simulink model "shuntDCmotor"  (R2018a)
settings: Solver=VariableStepAuto  StartTime=0.0  StopTime=10  RelTol=1e-3
values from neighbouring files (symbols this model uses):
  Bm = 0.00000604    (= 6.04e-06)    [PMDCparameters.m]    (also in SEDCparameters.m = 1.074e-06; SeriseDCparameters.m = 0.0025; ShuntDCparameters.m = 1.074e-06)
  J = 0.00000161    (= 1.61e-06)    [PMDCparameters.m]    (also in SEDCparameters.m = 0.21; SeriseDCparameters.m = 0.02365; ShuntDCparameters.m = 0.21)
  LAA = 0.12    [PMDCparameters.m]    (also in SEDCparameters.m = 0.01; SeriseDCparameters.m; ShuntDCparameters.m = 0.01)
  LAF = 0.004    [SEDCparameters.m]    (also in SeriseDCparameters.m = 0.0675; ShuntDCparameters.m)
  LFF = 0.167    [SEDCparameters.m]    (also in SeriseDCparameters.m = 0.03; ShuntDCparameters.m)
  ra = 7    [PMDCparameters.m]    (also in SEDCparameters.m = 0.013; SeriseDCparameters.m = 1.5; ShuntDCparameters.m = 0.013)
  rf = 1.43    [SEDCparameters.m]    (also in SeriseDCparameters.m = 0.7; ShuntDCparameters.m)
  Tl = 0.003    [PMDCparameters.m]    (also in SEDCparameters.m = 2.493; SeriseDCparameters.m = 10; ShuntDCparameters.m = 2.493)
  Va = 6    [PMDCparameters.m]    (also in SEDCparameters.m = 24; SeriseDCparameters.m = 100; ShuntDCparameters.m = 24)
libraries: fl_lib x15, nesl_utility x10, powerlib x3
settings Model: Creator=Noor  LastModifiedBy=Noor

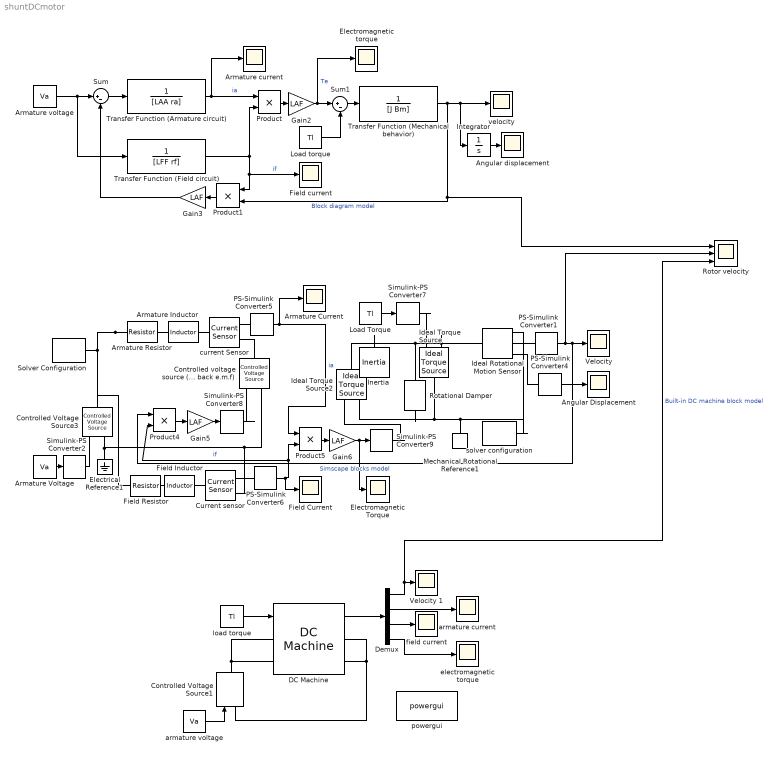
== system shuntDCmotor ==
  " Ideal Torque Source" : fl_lib/Mechanical/Mechanical Sources/Ideal Torque Source
  Angular Displacement : Scope
  Angular displacement : Scope
  Armature Voltage : Constant  Value=Va
  Armature Inductor : fl_lib/Electrical/Electrical Elements/Inductor  l=LAA H  r=0 Ohm  g=0 1/Ohm  i_specify=off  i_priority=None  i=0 A  i_nominal_specify=off  i_nominal_unit=A  i_nominal_value=1  v_specify=off  v_priority=None  v=0 V  v_nominal_specify=off  v_nominal_unit=V  v_nominal_value=1  i_L_specify=off  i_L_priority=High  i_L=0 A  i_L_nominal_specify=off  i_L_nominal_unit=A  i_L_nominal_value=1
  Armature Resistor : fl_lib/Electrical/Electrical Elements/Resistor  R=ra Ohm  i_specify=off  i_priority=None  i=0 A  i_nominal_specify=off  i_nominal_unit=A  i_nominal_value=1  v_specify=off  v_priority=None  v=0 V  v_nominal_specify=off  v_nominal_unit=V  v_nominal_value=1
  Armature Current : Scope
  Armature current : Scope
  Armature voltage : Constant  Value=Va
  Controlled voltage source (i.e. back e.m.f) : fl_lib/Electrical/Electrical Sources/Controlled Voltage Source
  Controlled Voltage Source3 : fl_lib/Electrical/Electrical Sources/Controlled Voltage Source
  Controlled Voltage Source1 : powerlib/Electrical Sources/Controlled Voltage Source  Initialize=on  Source_Type=AC  Amplitude=0  Phase=0  Frequency=0  Measurements=None
  Current sensor : fl_lib/Electrical/Electrical Sensors/Current Sensor
  DC Machine : powerlib/Machines/DC Machine  PresetModel=No  MechanicalLoad=Torque TL  FieldType=Wound  ShowDetailedParameters=on  MeasurementBus=off  RLa=[ra LAA]  RLf=[rf LFF]  Laf=LAF  MachineConstant=Torque constant (N.m/A)  Ke=1.8  Kt=1.8  J=J  Bm=Bm  Tf=0  w0=0  Ifinit=0  TsPowergui=0  TsBlock=-1
  Demux : Demux
  Electrical Reference1 : fl_lib/Electrical/Electrical Elements/Electrical Reference
  Electromagnetic Torque : Scope
  Electromagnetic torque : Scope
  Field Inductor : fl_lib/Electrical/Electrical Elements/Inductor  l=LFF H  r=0 Ohm  g=0 1/Ohm  i_specify=off  i_priority=None  i=0 A  i_nominal_specify=off  i_nominal_unit=A  i_nominal_value=1  v_specify=off  v_priority=None  v=0 V  v_nominal_specify=off  v_nominal_unit=V  v_nominal_value=1  i_L_specify=off  i_L_priority=High  i_L=0 A  i_L_nominal_specify=off  i_L_nominal_unit=A  i_L_nominal_value=1
  Field Resistor : fl_lib/Electrical/Electrical Elements/Resistor  R=rf Ohm  i_specify=off  i_priority=None  i=0 A  i_nominal_specify=off  i_nominal_unit=A  i_nominal_value=1  v_specify=off  v_priority=None  v=0 V  v_nominal_specify=off  v_nominal_unit=V  v_nominal_value=1
  Field Current : Scope
  Field current : Scope
  Gain{2..3,5..6} (4 alike) : Gain  Gain=LAF
  Ideal Rotational Motion Sensor : fl_lib/Mechanical/Mechanical Sensors/Ideal Rotational Motion Sensor  offset=0 rev
  Ideal Torque Source2 : fl_lib/Mechanical/Mechanical Sources/Ideal Torque Source
  "Inertia " : fl_lib/Mechanical/Rotational Elements/Inertia  inertia=J kg*m^2  w_specify=off  w_priority=High  w=0 rad/s  w_nominal_specify=off  w_nominal_unit=rad/s  w_nominal_value=1  t_specify=off  t_priority=None  t=0 N*m  t_nominal_specify=off  t_nominal_unit=N*m  t_nominal_value=1
  Integrator : Integrator
  Load Torque : Constant  Value=Tl
  Load torque : Constant  Value=Tl
  Mechanical Rotational Reference1 : fl_lib/Mechanical/Rotational Elements/Mechanical Rotational Reference
  PS-Simulink Converter{1,4..6} (4 alike) : nesl_utility/PS-Simulink Converter  PhysicalDomain=network_engine_domain  SubClassName=ps_output  LeftPortType=input  RightPortType=output  PseudoPeriodic=off  Frequencies=[]  Unit=1  AffineConversion=off
  Product{,1,4..5} (4 alike) : Product
  "Rotational Damper  " : fl_lib/Mechanical/Rotational Elements/Rotational Damper  D=Bm N*m/(rad/s)  w_specify=off  w_priority=None  w=0 rad/s  w_nominal_specify=off  w_nominal_unit=rad/s  w_nominal_value=1  t_specify=off  t_priority=None  t=0 N*m  t_nominal_specify=off  t_nominal_unit=N*m  t_nominal_value=1
  Rotor velocity : Scope  NumInputPorts=3
  Simulink-PS Converter{2,7..9} (4 alike) : nesl_utility/Simulink-PS Converter  PhysicalDomain=network_engine_domain  SubClassName=ps_input  LeftPortType=input  RightPortType=output  PseudoPeriodic=off  Frequencies=[]  NoiseDistribution=none  NoiseParameters=[]  Unit=1  AffineConversion=off  FilteringAndDerivatives=provide  SimscapeFilterOrder=1  InputFilterTimeConstant=0.001  UdotUserProvided=0
  Solver Configuration : nesl_utility/Solver Configuration  PhysicalDomain=network_engine_domain  SubClassName=solver  LeftPortType=input  RightPortType=generic  Tones=[]  Harmonics=[]  SimulateNoise=off  Profile=off  UseLocalSampling=off  EnableSwitchedLinearOptims=on  FrequencyDomain=off  UseCCode=off  RelTol=0.001  AbsTol=1e-06  MinStep=1e-09  ToWorkspace=off  RevertToSquareIcSolve=off  NumHomotopyIterations=100  PhasorMode=off  PhasorModeNumHarmonics=1  DoDC=off  ResidualTolerance=1e-09  UseLocalSolver=off  LocalSolverChoice=NE_BACKWARD_EULER_ADVANCER  LocalSolverSampleTime=0.001  DoFixedCost=off  MaxNonlinIter=3  MaxModeIter=2  LinearAlgebra=Sparse  EquationFormulation=NE_TIME_EF  DelaysMemoryBudget=1024  AutomaticFiltering=on  FilteringTimeConstant=0.001
  Sum : Sum  Inputs=|+-
  Sum1 : Sum  Inputs=|+-
  Transfer Function (Armature circuit) : TransferFcn  Denominator=[LAA ra]
  Transfer Function (Field circuit) : TransferFcn  Denominator=[LFF rf]
  Transfer Function (Mechanical behavior) : TransferFcn  Denominator=[J Bm]
  Velocity : Scope
  Velocity 1 : Scope
  armature current : Scope
  armature voltage : Constant  Value=Va
  "current Sensor " : fl_lib/Electrical/Electrical Sensors/Current Sensor
  "electromagnetic torque " : Scope
  field current : Scope
  load torque : Constant  Value=Tl
  powergui : powerlib/powergui  Priority=1  SimulationMode=Continuous  SampleTime=50e-6  frequency=60  Iterations=50  frequencyindice=0  Pbase=100e6  ErrMax=1e-4  UnitsV=kV  UnitsW=MW  buscounter=0  FunctionMessages=off  echomessages=off  EnableUseOfTLC=off  CurrentSourceSwitches=off  DisableSnubberDevices=off  DisableRonSwitches=off  DisableVfSwitches=off  DisplayEquations=off  SolverType=Tustin/Backward Euler (TBE)  Interpol=off  ExternalGateDelay=off  methode=off  Ts=100  x0status=blocks  SPID=on  SwTol=0  HookPort=off  RestoreLinks=warning  ResistiveCurrentMeasurement=off  Frange=[0:2:500]  Ylog=off  Xlog=on  ShowGrid=off  save=off  variable=ZData  structure=0  ZoomFFT=off  StartTime=0.0  cycles=1  DisplayStyle=1  fundamental=60  FreqAxis=off  MaxFrequency=1000  frequencyindicesteady=1  RmsSteady=1  display=off
  solver configuration : nesl_utility/Solver Configuration  PhysicalDomain=network_engine_domain  SubClassName=solver  LeftPortType=input  RightPortType=generic  Tones=[]  Harmonics=[]  SimulateNoise=off  Profile=off  UseLocalSampling=off  EnableSwitchedLinearOptims=on  FrequencyDomain=off  UseCCode=off  RelTol=0.001  AbsTol=1e-06  MinStep=1e-09  ToWorkspace=off  RevertToSquareIcSolve=off  NumHomotopyIterations=100  PhasorMode=off  PhasorModeNumHarmonics=1  DoDC=off  ResidualTolerance=1e-09  UseLocalSolver=off  LocalSolverChoice=NE_BACKWARD_EULER_ADVANCER  LocalSolverSampleTime=0.001  DoFixedCost=off  MaxNonlinIter=3  MaxModeIter=2  LinearAlgebra=Sparse  EquationFormulation=NE_TIME_EF  DelaysMemoryBudget=1024  AutomaticFiltering=on  FilteringTimeConstant=0.001
  velocity : Scope
  wires:
  Transfer Function (Mechanical behavior)/1 -> Rotor velocity/1, Product1/2, Integrator/1, velocity/1  "Block diagram model"
  Gain2/1 -> Electromagnetic torque/1, Sum1/1  "Te"
  Gain3/1 -> Sum/2
  Sum/1 -> Transfer Function (Armature circuit)/1
  Armature voltage/1 -> Transfer Function (Field circuit)/1, Sum/1
  Transfer Function (Armature circuit)/1 -> Armature current/1, Product/1  "ia"
  Transfer Function (Field circuit)/1 -> Field current/1, Product1/1, Product/2  "if"
  Product1/1 -> Gain3/1
  Sum1/1 -> Transfer Function (Mechanical behavior)/1
  Product/1 -> Gain2/1
  Demux/3 -> field current/1
  Demux/1 -> Rotor velocity/3, Velocity 1/1  "Built-in DC machine block model"
  Demux/4 -> "electromagnetic torque "/1
  DC Machine/1 -> Demux/1
  Demux/2 -> armature current/1
  armature voltage/1 -> Controlled Voltage Source1/1
  load torque/1 -> DC Machine/1
  PS-Simulink Converter4/1 -> Angular Displacement/1
  Armature Voltage/1 -> Simulink-PS Converter2/1
  Product5/1 -> Gain6/1
  Product4/1 -> Gain5/1
  PS-Simulink Converter1/1 -> Rotor velocity/2, Product4/1, Velocity/1  "Simscape blocks model"
  Load Torque/1 -> Simulink-PS Converter7/1
  PS-Simulink Converter5/1 -> Armature Current/1, Product5/1  "ia"
  Gain6/1 -> Electromagnetic Torque/1, Simulink-PS Converter9/1
  Gain5/1 -> Simulink-PS Converter8/1
  PS-Simulink Converter6/1 -> Product5/2, Product4/2, Field Current/1  "if"
  Integrator/1 -> Angular displacement/1
  Load torque/1 -> Sum1/2
  connections:
  Controlled Voltage Source1/RConn1 -- DC Machine/LConn2 -- DC Machine/LConn1
  Controlled Voltage Source1/LConn1 -- DC Machine/RConn2 -- DC Machine/RConn1
  " Ideal Torque Source"/RConn2 -- Ideal Torque Source2/LConn1 -- "Inertia "/LConn1 -- "Rotational Damper  "/LConn1 -- Ideal Rotational Motion Sensor/LConn1
  " Ideal Torque Source"/LConn1 -- "Rotational Damper  "/RConn1 -- Ideal Torque Source2/RConn2 -- Ideal Rotational Motion Sensor/RConn1 -- solver configuration/RConn1 -- Mechanical Rotational Reference1/LConn1
  Controlled voltage source (i.e. back e.m.f)/RConn2 -- Current sensor/RConn2 -- Controlled Voltage Source3/RConn2 -- Electrical Reference1/LConn1
  Armature Resistor/LConn1 -- Field Resistor/LConn1 -- Controlled Voltage Source3/LConn1 -- Solver Configuration/RConn1
  PS-Simulink Converter4/LConn1 -- Ideal Rotational Motion Sensor/RConn3
  Controlled voltage source (i.e. back e.m.f)/LConn1 -- "current Sensor "/RConn2
  PS-Simulink Converter1/LConn1 -- Ideal Rotational Motion Sensor/RConn2
  Simulink-PS Converter9/RConn1 -- Ideal Torque Source2/RConn1
  PS-Simulink Converter5/LConn1 -- "current Sensor "/RConn1
  Field Inductor/LConn1 -- Field Resistor/RConn1
  Simulink-PS Converter8/RConn1 -- Controlled voltage source (i.e. back e.m.f)/RConn1
  Simulink-PS Converter7/RConn1 -- " Ideal Torque Source"/RConn1
  Armature Inductor/LConn1 -- Armature Resistor/RConn1
  Controlled Voltage Source3/RConn1 -- Simulink-PS Converter2/RConn1
  "current Sensor "/LConn1 -- Armature Inductor/RConn1
  PS-Simulink Converter6/LConn1 -- Current sensor/RConn1
  Current sensor/LConn1 -- Field Inductor/RConn1
